simulink library "EnergyStorage"  (R2023a)
settings: Solver=VariableStepAuto  StartTime=0.0  StopTime=10.0  RelTol=1e-3
undefined symbols (not defined in the file or in its folder): batterymodel, h, H_u, k_cs, Q_SC_IC, rho_f
libraries: simulink x2
settings Model: Creator=dadikozyanaa  LastModifiedBy=bestt
settings DebuggingCC: UnconnectedInputMsg=warning  UnconnectedOutputMsg=warning  UnconnectedLineMsg=warning
settings ModelReferenceCC: EnableRefExpFcnMdlSchedulingChecks=on
settings RTWCC: DLArmComputeVersion=19.05

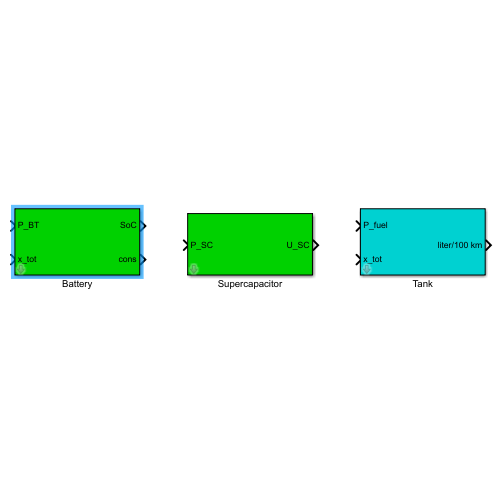
[thumbnail: Simulink's stored preview of the top-level diagram]
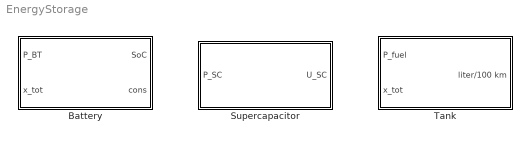
== system EnergyStorage ==
  Battery : Subsystem  mask(Battery){init_SoC=50, bt_Np=1, bt_Ns=1, SoC_low=10, SoC_high=90, bt_cap=0.018838, bt_vol=3.425, batnumberSim=1}
      mask prompts: init_SoC "Initial SoC [%]:"; bt_Np "Number of cells connected in parallel [-]:"; bt_Ns "Number of cells connected in series [-]:"; SoC_low "Lower SoC bound [%]"; SoC_high "Upper SoC bound [%]"; bt_cap "Battery pack capacity [kWh]:"; bt_vol "Battery pack voltage [V]:"; batnumberSim "Only for auto"
      mask help:
      | This block simulates a battery.
      |
      | Data:
      | ====
      | 	5.5	Nominal cell capacity [Ah]
      | 	3.425	Nominal cell voltage [V]
      |
      | Input:
      | =====
      | 	P_BT	Power from/to battery [W]
      | 	x_tot	Total distance [m]
      |
      | Output:
      | =====
      | 	SoC	Battery state of charge [%]
      | 	cons	Energy consumption [kWh/100km]
      |
      | Update the battery capacity only by scaling it with number of cells connected in series and parallel.
      mask init:
      | init_BT;
      mask Callback bt_Np:
      | Ns = str2num(get_param(gcb,'bt_Ns'));
      | Np = str2num(get_param(gcb,'bt_Np'));
      | 
      | %set_param(gcb,'bt_cap',num2str(Np*Ns*5.5*3.425*1e-3));
      | %set_param(gcb,'bt_vol',num2str(Ns*3.425));
      | 
      | p = Simulink.Mask.get(gcb);
      | cap = p.Parameters(6);
      | vol = p.Parameters(7);
      | 
      | cap.Enabled = 'on';
      | cap.Value = num2str(Np*Ns*5.5*3.425*1e-3);
      | cap.Enabled = 'off';
      | 
      | vol.Enabled = 'on';
      | vol.Value = num2str(Ns*3.425);
      | vol.Enabled = 'off';
      mask Callback bt_Ns:
      | Ns = str2num(get_param(gcb,'bt_Ns'));
      | Np = str2num(get_param(gcb,'bt_Np'));
      | 
      | %set_param(gcb,'bt_cap',num2str(Np*Ns*5.5*3.425*1e-3));
      | %set_param(gcb,'bt_vol',num2str(Ns*3.425));
      | 
      | p = Simulink.Mask.get(gcb);
      | cap = p.Parameters(6);
      | vol = p.Parameters(7);
      | 
      | cap.Enabled = 'on';
      | cap.Value = num2str(Np*Ns*5.5*3.425*1e-3);
      | cap.Enabled = 'off';
      | 
      | vol.Enabled = 'on';
      | vol.Value = num2str(Ns*3.425);
      | vol.Enabled = 'off';
      mask DialogControl Container3 Prompt: Read only
  Supercapacitor : Subsystem  Tag=supercap  mask(Supercapacitor){C_SC=8, R_SC=0.72, U_SC_max=225, P_SC_max=17500, Q_SC_IC_rel=95, N_SC=6}
      mask prompts: C_SC "Capacity of each supercap [F]"; R_SC "Internal resistance of each supercap [Ohm]"; U_SC_max "Maximum voltage of each supercap  [V]"; P_SC_max "Maximum power of each supercap [W]"; Q_SC_IC_rel "Initial charge of each supercap [%]"; N_SC "Number of supercaps (parallel connection) [-]"
      mask help:
      | The supercap is a fast electric energy buffer.
      |
      | Input:
      | =====
      | 	P_SC	Power to/from the supercap [W]
      | 		P_SC < 0: SC charging
      | 		P_SC > 0: SC discharging
      |
      | Output:
      | ======
      | 	U_SC	Voltage of the supercap [V]
      mask init:
      | init_SC;
  Tank : Subsystem  Tag=tank  mask(Tank){fuel=Gasoline, flag_cold_start=on}
      mask prompts: flag_cold_start "Include cold start losses"
      mask help:
      | This block integrates the power (the fuel mass flow) required by the combustion engine or the fuel cell and calculates the energy consumption in liter/100 km.
      |
      | Input:
      | =====
      | 	P_fuel	Power (fuel mass flow) required [W]
      | 	x_tot	Total distance [m]
      |
      | Output:
      | ======
      | 	V	Fuel consumption [liter/100 km]
      mask init:
      | init_tank;
      mask TypeOptions fuel: Gasoline | Diesel | Hydrogen

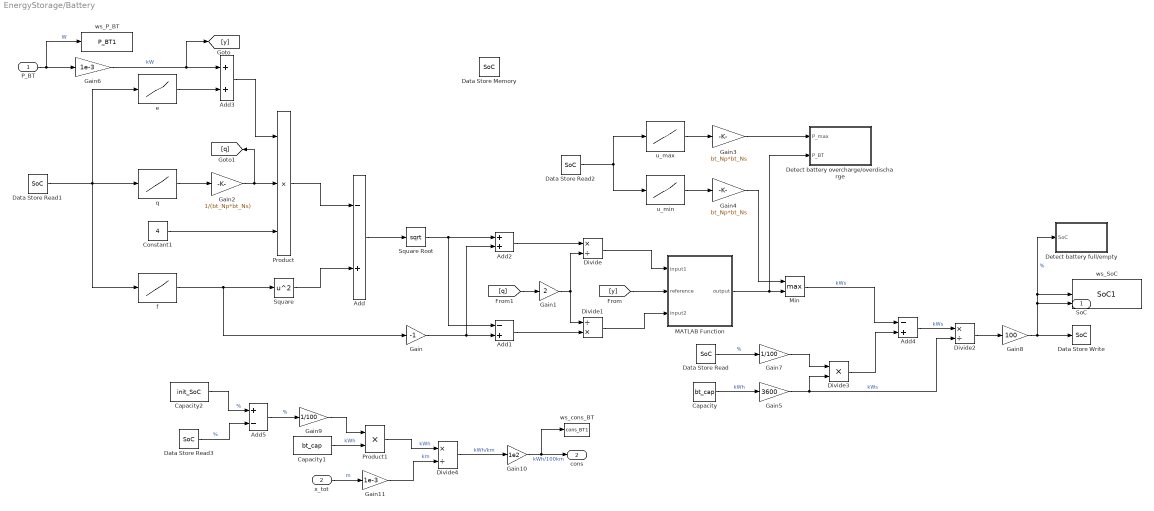
== system EnergyStorage/Battery ==
  P_BT : Inport
  x_tot : Inport  Port=2
  Add : Sum  Inputs=-+
  Add1 : Sum  Inputs=-+
  Add2 : Sum
  Add3 : Sum
  Add4 : Sum  Inputs=-+
  Add5 : Sum  Inputs=+-
  Capacity : Constant  Value=bt_cap
  Capacity1 : Constant  Value=bt_cap
  Capacity2 : Constant  Value=init_SoC
  Constant1 : Constant  Value=4
  Data Store Memory : DataStoreMemory  DataStoreName=SoC  ReadBeforeWriteMsg=warning  WriteAfterWriteMsg=warning  WriteAfterReadMsg=warning  InitialValue=init_SoC  ShowAdditionalParam=off  OutMin=0  OutMax=100
  Data Store Read{,1..3} (4 alike) : DataStoreRead  DataStoreName=SoC  IndexOptions=Index vector (dialog)  Indices=1  OutputSizes=1
  Data Store Write : DataStoreWrite  DataStoreName=SoC  IndexOptions=Index vector (dialog)  Indices=1  OutputSizes=1
  Detect battery full/empty : Subsystem
  Detect battery overcharge/overdischarge : Subsystem
  Divide : Product  Inputs=*/
  Divide1 : Product  Inputs=/*
  Divide2 : Product  Inputs=*/
  Divide3 : Product  Inputs=**
  Divide4 : Product  Inputs=*/
  Gain : Gain  Gain=-1
  Gain1 : Gain  Gain=2
  Gain10 : Gain  Gain=1e2
  Gain11 : Gain  Gain=1e-3
  Gain2 : Gain  Gain=1/(bt_Np*bt_Ns)
  Gain3 : Gain  Gain=bt_Np*bt_Ns
  Gain4 : Gain  Gain=bt_Np*bt_Ns
  Gain5 : Gain  Gain=3600
  Gain6 : Gain  Gain=1e-3
  Gain7 : Gain  Gain=1/100
  Gain8 : Gain  Gain=100
  Gain9 : Gain  Gain=1/100
  MATLAB Function : MATLAB Function  TreatAsAtomicUnit=on
  Min : MinMax  Function=max  Inputs=2
  Product : Product  Inputs=3
  Product1 : Product
  Square : Math  Operator=square
  Square Root : Sqrt
  e : Lookup  InputValues=batterymodel.qfe_SoC  Table=batterymodel.e
  f : Lookup  InputValues=batterymodel.qfe_SoC  Table=batterymodel.f
  q : Lookup  InputValues=batterymodel.qfe_SoC  Table=batterymodel.q
  u_max : Lookup  InputValues=batterymodel.u_max_SoC  Table=batterymodel.u_max
  u_min : Lookup  InputValues=batterymodel.u_min_SoC  Table=batterymodel.u_min
  ws_P_BT : ToWorkspace  VariableName=P_BT1  SampleTime=-1
  ws_SoC : ToWorkspace  VariableName=SoC1  SampleTime=-1
  ws_cons_BT : ToWorkspace  VariableName=cons_BT1  SampleTime=-1
  SoC : Outport
  cons : Outport  Port=2
  wires:
  Gain9/1 -> Product1/1
  Gain7/1 -> Divide3/1
  Add5/1 -> Gain9/1  "%"
  Min/1 -> Add4/1  "kWs"
  Data Store Read/1 -> Gain7/1  "%"
  Data Store Read2/1 -> u_max/1, u_min/1
  [q] -> Gain1/1
  Divide1/1 -> MATLAB Function/3(input2)
  Gain8/1 -> Data Store Write/1, Detect battery full/empty/1(SoC), ws_SoC/1, SoC/1  "%"
  P_BT/1 -> ws_P_BT/1, Gain6/1  "W"
  u_max/1 -> Gain3/1
  Gain11/1 -> Divide4/2  "km"
  Gain10/1 -> ws_cons_BT/1, cons/1  "kWh/100km"
  Divide4/1 -> Gain10/1  "kWh/km"
  Gain/1 -> Add2/2, Add1/2
  Gain2/1 -> [q], Product/2
  Add4/1 -> Divide2/1  "kWs"
  Gain4/1 -> Min/1
  Gain3/1 -> Detect battery overcharge/overdischarge/1(P_max)
  Add/1 -> Square Root/1
  Data Store Read3/1 -> Add5/2  "%"
  u_min/1 -> Gain4/1
  Data Store Read1/1 -> f/1, e/1, q/1
  Divide2/1 -> Gain8/1
  x_tot/1 -> Gain11/1  "m"
  Product1/1 -> Divide4/1  "kWh"
  MATLAB Function/1(output) -> Detect battery overcharge/overdischarge/2(P_BT), Min/2
  q/1 -> Gain2/1
  Divide3/1 -> Add4/2
  [y] -> MATLAB Function/2(reference)
  Capacity1/1 -> Product1/2  "kWh"
  Divide/1 -> MATLAB Function/1(input1)
  Add3/1 -> Product/1
  e/1 -> Add3/2
  Gain1/1 -> Divide1/1, Divide/2
  Capacity/1 -> Gain5/1  "kWh"
  Add2/1 -> Divide/1
  Square/1 -> Add/2
  Capacity2/1 -> Add5/1  "%"
  Add1/1 -> Divide1/2
  Gain5/1 -> Divide3/2, Divide2/2  "kWs"
  Product/1 -> Add/1
  Constant1/1 -> Product/3
  f/1 -> Gain/1, Square/1
  Gain6/1 -> [y], Add3/1  "kW"
  Square Root/1 -> Add1/1, Add2/1

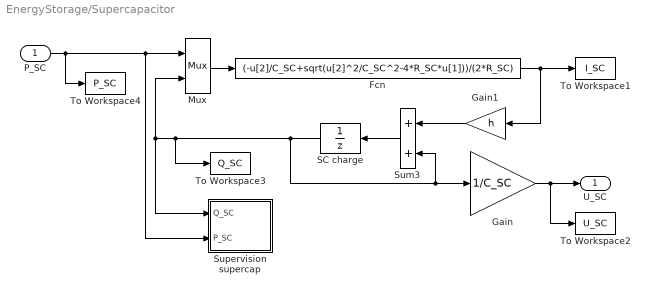
== system EnergyStorage/Supercapacitor ==
  P_SC : Inport
  Fcn : Fcn  Expr=(-u[2]/C_SC+sqrt(u[2]^2/C_SC^2-4*R_SC*u[1]))/(2*R_SC)
  Gain : Gain  Gain=1/C_SC  SaturateOnIntegerOverflow=on  OutDataTypeStr=Inherit: Same as input  ParamDataTypeStr=Inherit: Same as input
  Gain1 : Gain  Gain=h  SaturateOnIntegerOverflow=on  OutDataTypeStr=Inherit: Same as input  ParamDataTypeStr=Inherit: Same as input
  Mux : Mux  Inputs=2
  SC charge : UnitDelay  InitialCondition=Q_SC_IC  SampleTime=h
  Sum3 : Sum  InputSameDT=on  SaturateOnIntegerOverflow=on  OutDataTypeStr=Inherit: Same as first input
  Supervision supercap : Subsystem
  To Workspace1 : ToWorkspace  VariableName=I_SC  SampleTime=1
  To Workspace2 : ToWorkspace  VariableName=U_SC  SampleTime=1
  To Workspace3 : ToWorkspace  VariableName=Q_SC  SampleTime=1
  To Workspace4 : ToWorkspace  VariableName=P_SC  SampleTime=1
  U_SC : Outport  InitialOutput=0
  wires:
  P_SC/1 -> Supervision supercap/2(P_SC), Mux/1, To Workspace4/1
  Gain/1 -> To Workspace2/1, U_SC/1
  Fcn/1 -> To Workspace1/1, Gain1/1
  SC charge/1 -> To Workspace3/1, Supervision supercap/1(Q_SC), Mux/2, Gain/1, Sum3/2
  Sum3/1 -> SC charge/1
  Mux/1 -> Fcn/1
  Gain1/1 -> Sum3/1

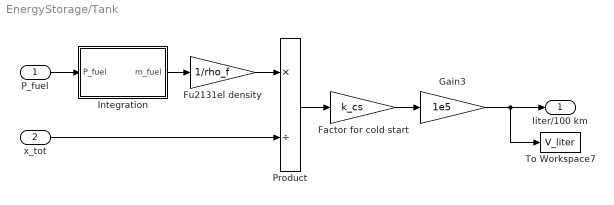
== system EnergyStorage/Tank ==
  P_fuel : Inport
  x_tot : Inport  Port=2
  Factor for cold start : Gain  Gain=k_cs  SaturateOnIntegerOverflow=on  OutDataTypeStr=Inherit: Same as input  ParamDataTypeStr=Inherit: Same as input
  Fu2131el density : Gain  Gain=1/rho_f  SaturateOnIntegerOverflow=on  OutDataTypeStr=Inherit: Same as input  ParamDataTypeStr=Inherit: Same as input
  Gain3 : Gain  Gain=1e5  SaturateOnIntegerOverflow=on  OutDataTypeStr=Inherit: Same as input  ParamDataTypeStr=Inherit: Same as input
  Integration : Subsystem
  Product : Product  Inputs=*/  InputSameDT=on  RndMeth=Zero  SaturateOnIntegerOverflow=on  OutDataTypeStr=Inherit: Same as first input
  To Workspace7 : ToWorkspace  VariableName=V_liter  SampleTime=-1
  liter/100 km : Outport  InitialOutput=0
  wires:
  P_fuel/1 -> Integration/1(P_fuel)
  x_tot/1 -> Product/2
  Integration/1(m_fuel) -> Fu2131el density/1
  Gain3/1 -> liter/100 km/1, To Workspace7/1
  Fu2131el density/1 -> Product/1
  Product/1 -> Factor for cold start/1
  Factor for cold start/1 -> Gain3/1

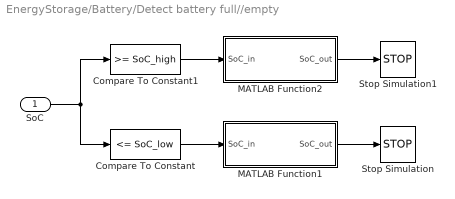
== system EnergyStorage/Battery/Detect battery full//empty ==
  SoC : Inport
  Compare To Constant : simulink/Logic and Bit Operations/Compare To Constant  relop=<=  const=SoC_low  OutDataTypeStr=boolean
  Compare To Constant1 : simulink/Logic and Bit Operations/Compare To Constant  relop=>=  const=SoC_high  OutDataTypeStr=boolean
  MATLAB Function1 : MATLAB Function  TreatAsAtomicUnit=on
  MATLAB Function2 : MATLAB Function  TreatAsAtomicUnit=on
  Stop Simulation : Stop
  Stop Simulation1 : Stop
  wires:
  Compare To Constant/1 -> MATLAB Function1/1(SoC_in)
  MATLAB Function1/1(SoC_out) -> Stop Simulation/1
  MATLAB Function2/1(SoC_out) -> Stop Simulation1/1
  Compare To Constant1/1 -> MATLAB Function2/1(SoC_in)
  SoC/1 -> Compare To Constant/1, Compare To Constant1/1

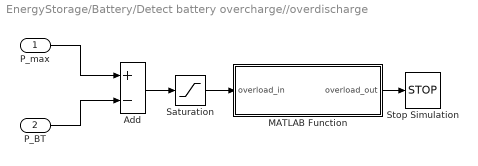
== system EnergyStorage/Battery/Detect battery overcharge//overdischarge ==
  P_max : Inport
  P_BT : Inport  Port=2
  Add : Sum  Inputs=+-
  MATLAB Function : MATLAB Function  TreatAsAtomicUnit=on
  Saturation : Saturate  UpperLimit=0  LowerLimit=-inf
  Stop Simulation : Stop
  wires:
  P_max/1 -> Add/1
  P_BT/1 -> Add/2
  Add/1 -> Saturation/1
  Saturation/1 -> MATLAB Function/1(overload_in)
  MATLAB Function/1(overload_out) -> Stop Simulation/1

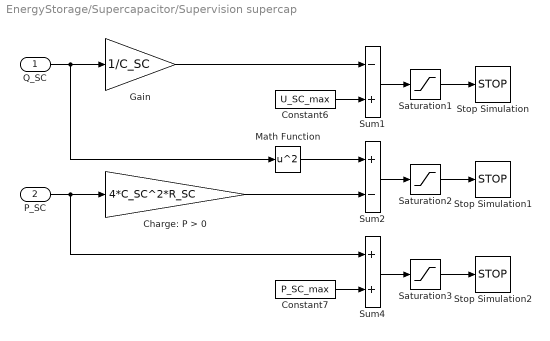
== system EnergyStorage/Supercapacitor/Supervision supercap ==
  Q_SC : Inport
  P_SC : Inport  Port=2
  Charge: P > 0 : Gain  Gain=4*C_SC^2*R_SC  SaturateOnIntegerOverflow=on  OutDataTypeStr=Inherit: Same as input  ParamDataTypeStr=Inherit: Same as input
  Constant6 : Constant  Value=U_SC_max
  Constant7 : Constant  Value=P_SC_max
  Gain : Gain  Gain=1/C_SC  SaturateOnIntegerOverflow=on  OutDataTypeStr=Inherit: Same as input  ParamDataTypeStr=Inherit: Same as input
  Math Function : Math  Operator=square  SignedPower=on
  Saturation1 : Saturate  UpperLimit=0  LowerLimit=-inf
  Saturation2 : Saturate  UpperLimit=0  LowerLimit=-inf
  Saturation3 : Saturate  UpperLimit=0  LowerLimit=-inf
  Stop Simulation : Stop
  Stop Simulation1 : Stop
  Stop Simulation2 : Stop
  Sum1 : Sum  Inputs=-+  InputSameDT=on  SaturateOnIntegerOverflow=on  OutDataTypeStr=Inherit: Same as first input
  Sum2 : Sum  Inputs=+-  InputSameDT=on  SaturateOnIntegerOverflow=on  OutDataTypeStr=Inherit: Same as first input
  Sum4 : Sum  InputSameDT=on  SaturateOnIntegerOverflow=on  OutDataTypeStr=Inherit: Same as first input
  wires:
  Math Function/1 -> Sum2/1
  Q_SC/1 -> Math Function/1, Gain/1
  Constant7/1 -> Sum4/2
  Constant6/1 -> Sum1/2
  Sum4/1 -> Saturation3/1
  Sum2/1 -> Saturation2/1
  Gain/1 -> Sum1/1
  Sum1/1 -> Saturation1/1
  Charge: P > 0/1 -> Sum2/2
  P_SC/1 -> Charge: P > 0/1, Sum4/1
  Saturation1/1 -> Stop Simulation/1
  Saturation2/1 -> Stop Simulation1/1
  Saturation3/1 -> Stop Simulation2/1

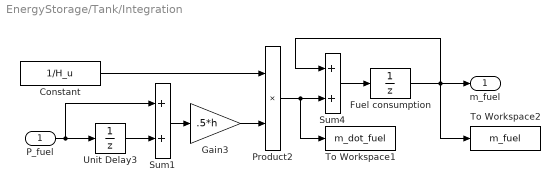
== system EnergyStorage/Tank/Integration ==
  P_fuel : Inport
  Constant : Constant  Value=1/H_u
  Fuel consumption : UnitDelay  SampleTime=h
  Gain3 : Gain  Gain=.5*h  SaturateOnIntegerOverflow=on  OutDataTypeStr=Inherit: Same as input  ParamDataTypeStr=Inherit: Same as input
  Product2 : Product  InputSameDT=on  RndMeth=Zero  SaturateOnIntegerOverflow=on  OutDataTypeStr=Inherit: Same as first input
  Sum1 : Sum  InputSameDT=on  SaturateOnIntegerOverflow=on  OutDataTypeStr=Inherit: Same as first input
  Sum4 : Sum  InputSameDT=on  SaturateOnIntegerOverflow=on  OutDataTypeStr=Inherit: Same as first input
  To Workspace1 : ToWorkspace  VariableName=m_dot_fuel  SampleTime=-1
  To Workspace2 : ToWorkspace  VariableName=m_fuel  SampleTime=-1
  Unit Delay3 : UnitDelay  SampleTime=h
  m_fuel : Outport  InitialOutput=0
  wires:
  Constant/1 -> Product2/1
  Gain3/1 -> Product2/2
  P_fuel/1 -> Sum1/1, Unit Delay3/1
  Unit Delay3/1 -> Sum1/2
  Sum1/1 -> Gain3/1
  Fuel consumption/1 -> m_fuel/1, Sum4/1, To Workspace2/1
  Sum4/1 -> Fuel consumption/1
  Product2/1 -> Sum4/2, To Workspace1/1

== matlab function EnergyStorage/Battery/Detect battery overcharge//overdischarge/MATLAB Function ==
  data: overload_in input; overload_out output
function overload_out = overload_fnc(overload_in)

if overload_in~=0
    disp('Simulation stopped due to Battery Overload.')
end

overload_out = overload_in;

== matlab function EnergyStorage/Battery/Detect battery full//empty/MATLAB Function2 ==
  data: SoC_in input; SoC_out output
function SoC_out = full(SoC_in)

if SoC_in~=0
    disp('Simulation stopped due to Battery Full.')
end

SoC_out = SoC_in;

== matlab function EnergyStorage/Battery/MATLAB Function ==
  data: input1 input; reference input; output output; input2 input
function output = fcn(input1,reference,input2)
if abs(input1) > 1.5*reference
    output = input2;
else
    output = input1;
end
end

== matlab function EnergyStorage/Battery/Detect battery full//empty/MATLAB Function1 ==
  data: SoC_in input; SoC_out output
function SoC_out = empty(SoC_in)

if SoC_in~=0
    disp('Simulation stopped due to Battery Empty.')
end

SoC_out = SoC_in;
